simulink model "iter_imas_contr_4"  (Simulink 8.5)
settings: Solver=ode1  StartTime=EqTime  StopTime=1e8  FixedStep=SimStep  MaxStep=5.e-3  MinStep=2e-4  RelTol=1.e-3
undefined symbols (not defined in the file): Elong, g1, g1_term, g2, g2_term, g3, g3_term, g4, g4_term, g5, g5_term, g6, g6_term, Imax, key_imas, n_gaps, n_mc, ncam, npf, ntur, RupRd, scr_data, SimStep, Vcspf_up, vec_imas, volt
libraries: simulink x56
(part 1 of 3)
settings Model: Creator=Kavin  ModifiedByFormat=Kavin  LastModifiedBy=Kavin  ExtModeTrigMode=oneshot  ExtModeArmWhenConnect=off  ExtModeAutoUpdateStatusClock=off
settings DataIOCC: LimitDataPoints=off  TimeSaveName=sim_time  SignalLoggingName=sigsOut
settings OptimizationCC: BooleanDataType=off  OptimizeBlockIOStorage=off  BufferReuse=off  GlobalBufferReuse=off  ExpressionFolding=off  ExpressionDepthLimit=128  LocalBlockOutputs=off  InitFltsAndDblsToZero=on
settings DebuggingCC: SaveWithParameterizedLinksMsg=none  SignalResolutionControl=TryResolveAllWithWarning  MultiTaskDSMMsg=warning  MultiTaskCondExecSysMsg=none  FcnCallInpInsideContextMsg=UseLocalSettings  StateNameClashWarn=none
settings HardwareCC: TargetUnknown=on
settings CodeAppCC: IgnoreCustomStorageClasses=off
settings GRTTargetCC: TargetFcnLib=ansi_tfl_tmw.mat

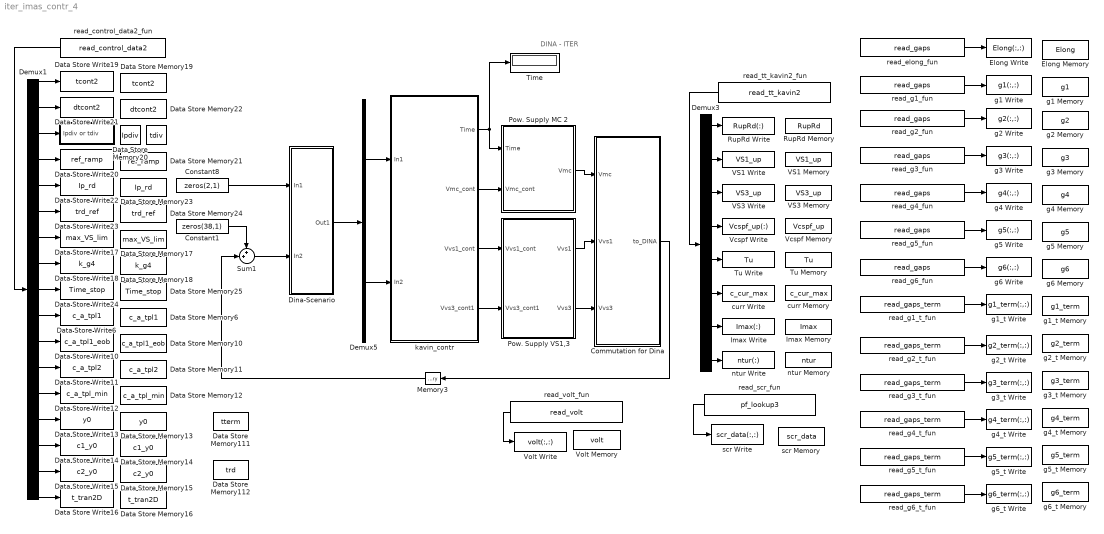
== system iter_imas_contr_4 ==
  note: DINA - ITER
  " " : DataStoreMemory  DataStoreName=tdiv  ReadBeforeWriteMsg=warning  WriteAfterWriteMsg=warning  WriteAfterReadMsg=warning  InitialValue=1e3
  "  " : Subsystem
  Commutation for Dina : Subsystem
  Constant1 : Constant  Value=zeros(38,1)
  Constant8 : Constant  Value=zeros(2,1)
  Data Store Memory10 : DataStoreMemory  DataStoreName=c_a_tpl1_eob  ReadBeforeWriteMsg=warning  WriteAfterWriteMsg=warning  WriteAfterReadMsg=warning
  Data Store Memory11 : DataStoreMemory  DataStoreName=c_a_tpl2  ReadBeforeWriteMsg=warning  WriteAfterWriteMsg=warning  WriteAfterReadMsg=warning
  Data Store Memory111 : DataStoreMemory  DataStoreName=tterm  ReadBeforeWriteMsg=warning  WriteAfterWriteMsg=warning  WriteAfterReadMsg=warning  InitialValue=1000
  Data Store Memory112 : DataStoreMemory  DataStoreName=trd  ReadBeforeWriteMsg=warning  WriteAfterWriteMsg=warning  WriteAfterReadMsg=warning  InitialValue=1000
  Data Store Memory12 : DataStoreMemory  DataStoreName=c_a_tpl_min  ReadBeforeWriteMsg=warning  WriteAfterWriteMsg=warning  WriteAfterReadMsg=warning
  Data Store Memory13 : DataStoreMemory  DataStoreName=y0  ReadBeforeWriteMsg=warning  WriteAfterWriteMsg=warning  WriteAfterReadMsg=warning
  Data Store Memory14 : DataStoreMemory  DataStoreName=c1_y0  ReadBeforeWriteMsg=warning  WriteAfterWriteMsg=warning  WriteAfterReadMsg=warning
  Data Store Memory15 : DataStoreMemory  DataStoreName=c2_y0  ReadBeforeWriteMsg=warning  WriteAfterWriteMsg=warning  WriteAfterReadMsg=warning
  Data Store Memory16 : DataStoreMemory  DataStoreName=t_tran2D  ReadBeforeWriteMsg=warning  WriteAfterWriteMsg=warning  WriteAfterReadMsg=warning
  Data Store Memory17 : DataStoreMemory  DataStoreName=max_VS_lim  ReadBeforeWriteMsg=warning  WriteAfterWriteMsg=warning  WriteAfterReadMsg=warning
  Data Store Memory18 : DataStoreMemory  DataStoreName=k_g4  ReadBeforeWriteMsg=warning  WriteAfterWriteMsg=warning  WriteAfterReadMsg=warning
  Data Store Memory19 : DataStoreMemory  DataStoreName=tcont2  ReadBeforeWriteMsg=warning  WriteAfterWriteMsg=warning  WriteAfterReadMsg=warning
  Data Store Memory20 : DataStoreMemory  DataStoreName=Ipdiv  ReadBeforeWriteMsg=warning  WriteAfterWriteMsg=warning  WriteAfterReadMsg=warning  InitialValue=0.1
  Data Store Memory21 : DataStoreMemory  DataStoreName=ref_ramp  ReadBeforeWriteMsg=warning  WriteAfterWriteMsg=warning  WriteAfterReadMsg=warning  InitialValue=1e-3
  Data Store Memory22 : DataStoreMemory  DataStoreName=dtcont2  ReadBeforeWriteMsg=warning  WriteAfterWriteMsg=warning  WriteAfterReadMsg=warning  InitialValue=1e-3
  Data Store Memory23 : DataStoreMemory  DataStoreName=Ip_rd  ReadBeforeWriteMsg=warning  WriteAfterWriteMsg=warning  WriteAfterReadMsg=warning
  Data Store Memory24 : DataStoreMemory  DataStoreName=trd_ref  ReadBeforeWriteMsg=warning  WriteAfterWriteMsg=warning  WriteAfterReadMsg=warning
  Data Store Memory25 : DataStoreMemory  DataStoreName=Time_stop  ReadBeforeWriteMsg=warning  WriteAfterWriteMsg=warning  WriteAfterReadMsg=warning
  Data Store Memory6 : DataStoreMemory  DataStoreName=c_a_tpl1  ReadBeforeWriteMsg=warning  WriteAfterWriteMsg=warning  WriteAfterReadMsg=warning
  Data Store Write10 : DataStoreWrite  DataStoreName=c_a_tpl1_eob  DataStoreElements=c_a_tpl1_eob
  Data Store Write11 : DataStoreWrite  DataStoreName=c_a_tpl2  DataStoreElements=c_a_tpl2
  Data Store Write12 : DataStoreWrite  DataStoreName=c_a_tpl_min  DataStoreElements=c_a_tpl_min
  Data Store Write13 : DataStoreWrite  DataStoreName=y0  DataStoreElements=y0
  Data Store Write14 : DataStoreWrite  DataStoreName=c1_y0  DataStoreElements=c1_y0
  Data Store Write15 : DataStoreWrite  DataStoreName=c2_y0  DataStoreElements=c2_y0
  Data Store Write16 : DataStoreWrite  DataStoreName=t_tran2D  DataStoreElements=t_tran2D
  Data Store Write17 : DataStoreWrite  DataStoreName=max_VS_lim  DataStoreElements=max_VS_lim
  Data Store Write18 : DataStoreWrite  DataStoreName=k_g4  DataStoreElements=k_g4
  Data Store Write19 : DataStoreWrite  DataStoreName=tcont2  DataStoreElements=tcont2
  Data Store Write20 : DataStoreWrite  DataStoreName=ref_ramp  DataStoreElements=ref_ramp
  Data Store Write21 : DataStoreWrite  DataStoreName=dtcont2  DataStoreElements=dtcont2
  Data Store Write22 : DataStoreWrite  DataStoreName=Ip_rd  DataStoreElements=Ip_rd
  Data Store Write23 : DataStoreWrite  DataStoreName=trd_ref  DataStoreElements=trd_ref
  Data Store Write24 : DataStoreWrite  DataStoreName=Time_stop  DataStoreElements=Time_stop
  Data Store Write6 : DataStoreWrite  DataStoreName=c_a_tpl1  DataStoreElements=c_a_tpl1
  Demux1 : Demux  Outputs=ones(1,17)
  Demux3 : Demux  Outputs=[6 1 1 11 1 1 11 12]
  Demux5 : Demux  Outputs=[15 123]
  Dina-Scenario : Subsystem
  Elong Memory : DataStoreMemory  DataStoreName=Elong  ReadBeforeWriteMsg=warning  WriteAfterWriteMsg=warning  WriteAfterReadMsg=warning  InitialValue=[0:49;zeros(1,50)]
  Elong Write : DataStoreWrite  DataStoreName=Elong  DataStoreElements=Elong(:,:)
  Imax Memory : DataStoreMemory  DataStoreName=Imax  ReadBeforeWriteMsg=warning  WriteAfterWriteMsg=warning  WriteAfterReadMsg=warning  InitialValue=ones(1,11)*1e6
  Imax Write : DataStoreWrite  DataStoreName=Imax  DataStoreElements=Imax(:)
  Memory3 : Memory
  Pow. Supply MC 2 : Subsystem
  Pow. Supply VS1,3 : Subsystem
  RupRd Memory : DataStoreMemory  DataStoreName=RupRd  ReadBeforeWriteMsg=warning  WriteAfterWriteMsg=warning  WriteAfterReadMsg=warning  InitialValue=[1; ones(3,1)*1e-6; -1e6; 1e-6]
  RupRd Write : DataStoreWrite  DataStoreName=RupRd  DataStoreElements=RupRd(:)
  Sum1 : Sum  Inputs=++|  SaturateOnIntegerOverflow=on  InputSameDT=on  OutDataTypeStr=Inherit: Same as first input
  Time : Display
  Tu Memory : DataStoreMemory  DataStoreName=Tu  ReadBeforeWriteMsg=warning  WriteAfterWriteMsg=warning  WriteAfterReadMsg=warning
  Tu Write : DataStoreWrite  DataStoreName=Tu  DataStoreElements=Tu
  VS1 Memory : DataStoreMemory  DataStoreName=VS1_up  ReadBeforeWriteMsg=warning  WriteAfterWriteMsg=warning  WriteAfterReadMsg=warning
  VS1 Write : DataStoreWrite  DataStoreName=VS1_up  DataStoreElements=VS1_up
  VS3 Memory : DataStoreMemory  DataStoreName=VS3_up  ReadBeforeWriteMsg=warning  WriteAfterWriteMsg=warning  WriteAfterReadMsg=warning
  VS3 Write : DataStoreWrite  DataStoreName=VS3_up  DataStoreElements=VS3_up
  Vcspf Memory : DataStoreMemory  DataStoreName=Vcspf_up  ReadBeforeWriteMsg=warning  WriteAfterWriteMsg=warning  WriteAfterReadMsg=warning  InitialValue=zeros(11,1)
  Vcspf Write : DataStoreWrite  DataStoreName=Vcspf_up  DataStoreElements=Vcspf_up(:)
  Volt Memory : DataStoreMemory  DataStoreName=volt  ReadBeforeWriteMsg=warning  WriteAfterWriteMsg=warning  WriteAfterReadMsg=warning  InitialValue=[(0:499);zeros(19,500)]
  Volt Write : DataStoreWrite  DataStoreName=volt  DataStoreElements=volt(:,:)
  curr Memory : DataStoreMemory  DataStoreName=c_cur_max  ReadBeforeWriteMsg=warning  WriteAfterWriteMsg=warning  WriteAfterReadMsg=warning
  curr Write : DataStoreWrite  DataStoreName=c_cur_max  DataStoreElements=c_cur_max
  g1 Memory : DataStoreMemory  DataStoreName=g1  ReadBeforeWriteMsg=warning  WriteAfterWriteMsg=warning  WriteAfterReadMsg=warning  InitialValue=[0:49;zeros(1,50)]
  g1 Write : DataStoreWrite  DataStoreName=g1  DataStoreElements=g1(:,:)
  g1_t Memory : DataStoreMemory  DataStoreName=g1_term  ReadBeforeWriteMsg=warning  WriteAfterWriteMsg=warning  WriteAfterReadMsg=warning  InitialValue=zeros(2, 50)
  g1_t Write : DataStoreWrite  DataStoreName=g1_term  DataStoreElements=g1_term(:,:)
  g2 Memory : DataStoreMemory  DataStoreName=g2  ReadBeforeWriteMsg=warning  WriteAfterWriteMsg=warning  WriteAfterReadMsg=warning  InitialValue=[0:49;zeros(1,50)]
  g2 Write : DataStoreWrite  DataStoreName=g2  DataStoreElements=g2(:,:)
  g2_t Memory : DataStoreMemory  DataStoreName=g2_term  ReadBeforeWriteMsg=warning  WriteAfterWriteMsg=warning  WriteAfterReadMsg=warning  InitialValue=zeros(2, 50)
  g2_t Write : DataStoreWrite  DataStoreName=g2_term  DataStoreElements=g2_term(:,:)
  g3 Memory : DataStoreMemory  DataStoreName=g3  ReadBeforeWriteMsg=warning  WriteAfterWriteMsg=warning  WriteAfterReadMsg=warning  InitialValue=[0:49;zeros(1,50)]
  g3 Write : DataStoreWrite  DataStoreName=g3  DataStoreElements=g3(:,:)
  g3_t Memory : DataStoreMemory  DataStoreName=g3_term  ReadBeforeWriteMsg=warning  WriteAfterWriteMsg=warning  WriteAfterReadMsg=warning  InitialValue=zeros(2, 50)
  g3_t Write : DataStoreWrite  DataStoreName=g3_term  DataStoreElements=g3_term(:,:)
  g4 Memory : DataStoreMemory  DataStoreName=g4  ReadBeforeWriteMsg=warning  WriteAfterWriteMsg=warning  WriteAfterReadMsg=warning  InitialValue=[0:49;zeros(1,50)]
  g4 Write : DataStoreWrite  DataStoreName=g4  DataStoreElements=g4(:,:)
  g4_t Memory : DataStoreMemory  DataStoreName=g4_term  ReadBeforeWriteMsg=warning  WriteAfterWriteMsg=warning  WriteAfterReadMsg=warning  InitialValue=zeros(2, 50)
  g4_t Write : DataStoreWrite  DataStoreName=g4_term  DataStoreElements=g4_term(:,:)
  g5 Memory : DataStoreMemory  DataStoreName=g5  ReadBeforeWriteMsg=warning  WriteAfterWriteMsg=warning  WriteAfterReadMsg=warning  InitialValue=[0:49;zeros(1,50)]
  g5 Write : DataStoreWrite  DataStoreName=g5  DataStoreElements=g5(:,:)
  g5_t Memory : DataStoreMemory  DataStoreName=g5_term  ReadBeforeWriteMsg=warning  WriteAfterWriteMsg=warning  WriteAfterReadMsg=warning  InitialValue=zeros(2, 50)
  g5_t Write : DataStoreWrite  DataStoreName=g5_term  DataStoreElements=g5_term(:,:)
  g6 Memory : DataStoreMemory  DataStoreName=g6  ReadBeforeWriteMsg=warning  WriteAfterWriteMsg=warning  WriteAfterReadMsg=warning  InitialValue=[0:49;zeros(1,50)]
  g6 Write : DataStoreWrite  DataStoreName=g6  DataStoreElements=g6(:,:)
  g6_t Memory : DataStoreMemory  DataStoreName=g6_term  ReadBeforeWriteMsg=warning  WriteAfterWriteMsg=warning  WriteAfterReadMsg=warning  InitialValue=zeros(2, 50)
  g6_t Write : DataStoreWrite  DataStoreName=g6_term  DataStoreElements=g6_term(:,:)
  kavin_contr : Subsystem
  ntur Memory : DataStoreMemory  DataStoreName=ntur  ReadBeforeWriteMsg=warning  WriteAfterWriteMsg=warning  WriteAfterReadMsg=warning  InitialValue="[554,554,554,554,554  248.6 115.2 185.9 169.9 216.8  459.4 1]"
  ntur Write : DataStoreWrite  DataStoreName=ntur  DataStoreElements=ntur(:)
  read_control_data2_fun : S-Function  FunctionName=read_control_data2  SFunctionModules=read_control_data2_wrapper read_control_data2
  read_elong_fun : S-Function  FunctionName=read_gaps  Parameters=0  SFunctionModules='read_gaps_wrapper read_gaps'
  read_g1_fun : S-Function  FunctionName=read_gaps  Parameters=1  SFunctionModules='read_gaps_wrapper read_gaps'
  read_g1_t_fun : S-Function  FunctionName=read_gaps_term  Parameters=1  SFunctionModules='read_gaps_term_wrapper read_gaps_term'
  read_g2_fun : S-Function  FunctionName=read_gaps  Parameters=2  SFunctionModules='read_gaps_wrapper read_gaps'
  read_g2_t_fun : S-Function  FunctionName=read_gaps_term  Parameters=2  SFunctionModules='read_gaps_term_wrapper read_gaps_term'
  read_g3_fun : S-Function  FunctionName=read_gaps  Parameters=3  SFunctionModules='read_gaps_wrapper read_gaps'
  read_g3_t_fun : S-Function  FunctionName=read_gaps_term  Parameters=3  SFunctionModules='read_gaps_term_wrapper read_gaps_term'
  read_g4_fun : S-Function  FunctionName=read_gaps  Parameters=4  SFunctionModules='read_gaps_wrapper read_gaps'
  read_g4_t_fun : S-Function  FunctionName=read_gaps_term  Parameters=4  SFunctionModules='read_gaps_term_wrapper read_gaps_term'
  read_g5_fun : S-Function  FunctionName=read_gaps  Parameters=5  SFunctionModules='read_gaps_wrapper read_gaps'
  read_g5_t_fun : S-Function  FunctionName=read_gaps_term  Parameters=5  SFunctionModules='read_gaps_term_wrapper read_gaps_term'
  read_g6_fun : S-Function  FunctionName=read_gaps  Parameters=6  SFunctionModules='read_gaps_wrapper read_gaps'
  read_g6_t_fun : S-Function  FunctionName=read_gaps_term  Parameters=6  SFunctionModules='read_gaps_term_wrapper read_gaps_term'
  read_scr_fun : S-Function  FunctionName=pf_lookup3  Parameters=1  SFunctionModules='pf_lookup3_wrapper read_pf'
  read_tt_kavin2_fun : S-Function  FunctionName=read_tt_kavin2  SFunctionModules=read_tt_kavin2_wrapper read_tt_kavin2
  read_volt_fun : S-Function  FunctionName=read_volt  Parameters=12  SFunctionModules='read_volt_wrapper read_volt'
  scr Memory : DataStoreMemory  DataStoreName=scr_data  ReadBeforeWriteMsg=warning  WriteAfterWriteMsg=warning  WriteAfterReadMsg=warning  InitialValue=[(0:499); zeros(12,500)]
  scr Write : DataStoreWrite  DataStoreName=scr_data  DataStoreElements=scr_data(:,:)
  wires:
  Demux5/1 -> kavin_contr/1(In1)
  Demux5/2 -> kavin_contr/2(In2)
  Dina-Scenario/1(Out1) -> Demux5/1
  Constant8/1 -> Dina-Scenario/1(In1)
  Constant1/1 -> Sum1/1
  Sum1/1 -> Dina-Scenario/2(In2)
  kavin_contr/2(Vmc_cont) -> Pow. Supply MC 2/2(Vmc_cont)
  Pow. Supply MC 2/1(Vmc) -> Commutation for Dina/1(Vmc)
  Commutation for Dina/1(to_DINA) -> Memory3/1
  read_tt_kavin2_fun/1 -> Demux3/1
  kavin_contr/3(Vvs1_cont) -> Pow. Supply VS1,3/1(Vvs1_cont)
  kavin_contr/4(Vvs3_cont1) -> Pow. Supply VS1,3/2(Vvs3_cont1)
  Pow. Supply VS1,3/2(Vvs3) -> Commutation for Dina/3(Vvs3)
  Pow. Supply VS1,3/1(Vvs1) -> Commutation for Dina/2(Vvs1)
  Demux3/8 -> ntur Write/1
  Demux3/7 -> Imax Write/1
  Demux3/6 -> curr Write/1
  Demux3/5 -> Tu Write/1
  Demux3/4 -> Vcspf Write/1
  Demux3/3 -> VS3 Write/1
  Demux3/2 -> VS1 Write/1
  Demux3/1 -> RupRd Write/1
  Memory3/1 -> Sum1/2
  read_elong_fun/1 -> Elong Write/1
  read_g1_fun/1 -> g1 Write/1
  read_g2_fun/1 -> g2 Write/1
  read_g3_fun/1 -> g3 Write/1
  read_g4_fun/1 -> g4 Write/1
  read_g5_fun/1 -> g5 Write/1
  read_g6_fun/1 -> g6 Write/1
  read_g1_t_fun/1 -> g1_t Write/1
  read_g2_t_fun/1 -> g2_t Write/1
  read_g3_t_fun/1 -> g3_t Write/1
  read_g4_t_fun/1 -> g4_t Write/1
  read_g5_t_fun/1 -> g5_t Write/1
  read_g6_t_fun/1 -> g6_t Write/1
  read_scr_fun/1 -> scr Write/1
  kavin_contr/1(Time) -> Time/1, Pow. Supply MC 2/1(Time)
  read_volt_fun/1 -> Volt Write/1
  read_control_data2_fun/1 -> Demux1/1
  Demux1/6 -> Data Store Write23/1
  Demux1/5 -> Data Store Write22/1
  Demux1/4 -> Data Store Write20/1
  Demux1/3 -> "  "/1("Ipdiv or tdiv ")
  Demux1/2 -> Data Store Write21/1
  Demux1/1 -> Data Store Write19/1
  Demux1/9 -> Data Store Write24/1
  Demux1/10 -> Data Store Write6/1
  Demux1/11 -> Data Store Write10/1
  Demux1/12 -> Data Store Write11/1
  Demux1/13 -> Data Store Write12/1
  Demux1/14 -> Data Store Write13/1
  Demux1/15 -> Data Store Write14/1
  Demux1/16 -> Data Store Write15/1
  Demux1/17 -> Data Store Write16/1
  Demux1/7 -> Data Store Write17/1
  Demux1/8 -> Data Store Write18/1

== system iter_imas_contr_4/   ==
  "Ipdiv or tdiv " : Inport
  Data Store Write19 : DataStoreWrite  DataStoreName=Ipdiv
  If : If  IfExpression=u1 >= 0  ShowElse=off
  If Action : Subsystem  TreatAsAtomicUnit=on
  wires:
  "Ipdiv or tdiv "/1 -> Data Store Write19/1, If Action/1("tdiv "), If/1
  If/1 -> If Action/Action

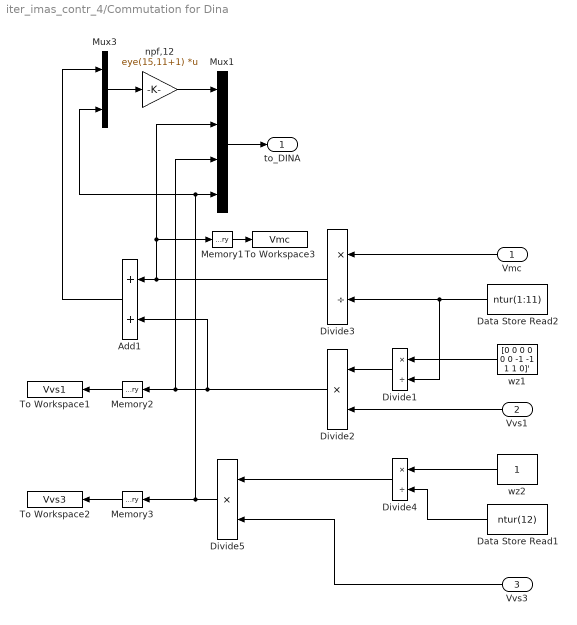
== system iter_imas_contr_4/Commutation for Dina ==
  Vmc : Inport
  Vvs1 : Inport  Port=2
  Vvs3 : Inport  Port=3
  Add1 : Sum
  Data Store Read1 : DataStoreRead  DataStoreName=ntur  DataStoreElements=ntur(12)
  Data Store Read2 : DataStoreRead  DataStoreName=ntur  DataStoreElements=ntur(1:11)
  Divide1 : Product  Inputs=*/
  Divide2 : Product  Inputs=**
  Divide3 : Product  Inputs=*/
  Divide4 : Product  Inputs=*/
  Divide5 : Product  Inputs=**
  Memory1 : Memory
  Memory2 : Memory
  Memory3 : Memory
  Mux1 : Mux
  Mux3 : Mux  Inputs=2
  To Workspace1 : ToWorkspace  VariableName=Vvs1
  To Workspace2 : ToWorkspace  VariableName=Vvs3
  To Workspace3 : ToWorkspace  VariableName=Vmc
  npf,12 : Gain  Gain=eye(15,11+1)  Multiplication=Matrix(K*u)
  wz1 : Constant  Value=[0 0 0 0 0 0 -1 -1 1 1 0]'
  wz2 : Constant
  to_DINA : Outport
  wires:
  Divide2/1 -> Add1/2, Mux1/3, Memory2/1
  Mux1/1 -> to_DINA/1
  Add1/1 -> Mux3/1
  Mux3/1 -> npf,12/1
  npf,12/1 -> Mux1/1
  Divide3/1 -> Add1/1, Mux1/2, Memory1/1
  Vmc/1 -> Divide3/1
  Data Store Read2/1 -> Divide1/2, Divide3/2
  wz1/1 -> Divide1/1
  Divide1/1 -> Divide2/1
  Vvs1/1 -> Divide2/2
  wz2/1 -> Divide4/1
  Data Store Read1/1 -> Divide4/2
  Divide4/1 -> Divide5/1
  Vvs3/1 -> Divide5/2
  Divide5/1 -> Mux3/2, Mux1/4, Memory3/1
  Memory1/1 -> To Workspace3/1
  Memory2/1 -> To Workspace1/1
  Memory3/1 -> To Workspace2/1

== system iter_imas_contr_4/Dina-Scenario ==
  In1 : Inport
  In2 : Inport  Port=2
  Constant15 : Constant  Value=zeros(54,1)
  Mux2 : Mux  Inputs=2
  S-Function1 : S-Function  FunctionName=dina_imas  Parameters=key_imas,vec_imas
  Terminator3 : Terminator
  To Workspace21 : ToWorkspace  VariableName=sim_shape
      settings: Decimation=DecimShape
  Out1 : Outport
  wires:
  In1/1 -> S-Function1/1
  S-Function1/2 -> Mux2/2
  S-Function1/3 -> To Workspace21/1
  S-Function1/4 -> Terminator3/1
  S-Function1/1 -> Mux2/1
  Mux2/1 -> Out1/1
  In2/1 -> S-Function1/2
  Constant15/1 -> S-Function1/3

== system iter_imas_contr_4/Pow. Supply MC 2 ==
  Time : Inport
  Vmc_cont : Inport  Port=2
  Difference : simulink/Discrete/Difference  ICPrevInput=0.0  InputProcessing=Inherited  OutMin=[]  OutMax=[]  OutDataType=sfix(16)  OutScaling=2^-10  DoSatur=off
  Pow. Supply MC 1 : Subsystem
  Vmc : Outport
  wires:
  Time/1 -> Difference/1
  Difference/1 -> Pow. Supply MC 1/1(dt)
  Pow. Supply MC 1/1(Vmc) -> Vmc/1
  Vmc_cont/1 -> Pow. Supply MC 1/2(Vmc_cont)

== system iter_imas_contr_4/Pow. Supply VS1,3 ==
  Vvs1_cont : Inport
  Vvs3_cont1 : Inport  Port=2
  Data Store Read1 : DataStoreRead  DataStoreName=VS1_up  DataStoreElements=VS1_up
  Data Store Read3 : DataStoreRead  DataStoreName=VS3_up  DataStoreElements=VS3_up
  Gain : Gain  Gain=-1
  Gain1 : Gain  Gain=-1
  Saturation Dynamic : simulink/Discontinuities/Saturation Dynamic  OutMin=[]  OutMax=[]  OutDataTypeStr=Inherit: Same as second input  OutDataType=fixdt(1, 16)  OutScaling=2^-10  DoSatur=off
  Saturation Dynamic1 : simulink/Discontinuities/Saturation Dynamic  OutMin=[]  OutMax=[]  OutDataTypeStr=Inherit: Same as second input  OutDataType=fixdt(1, 16)  OutScaling=2^-10  DoSatur=off
  Vvs1 : Outport
  Vvs3 : Outport  Port=2
  wires:
  Data Store Read1/1 -> Gain/1, Saturation Dynamic/1
  Gain/1 -> Saturation Dynamic/3
  Vvs1_cont/1 -> Saturation Dynamic/2
  Gain1/1 -> Saturation Dynamic1/3
  Data Store Read3/1 -> Gain1/1, Saturation Dynamic1/1
  Vvs3_cont1/1 -> Saturation Dynamic1/2
  Saturation Dynamic/1 -> Vvs1/1
  Saturation Dynamic1/1 -> Vvs3/1

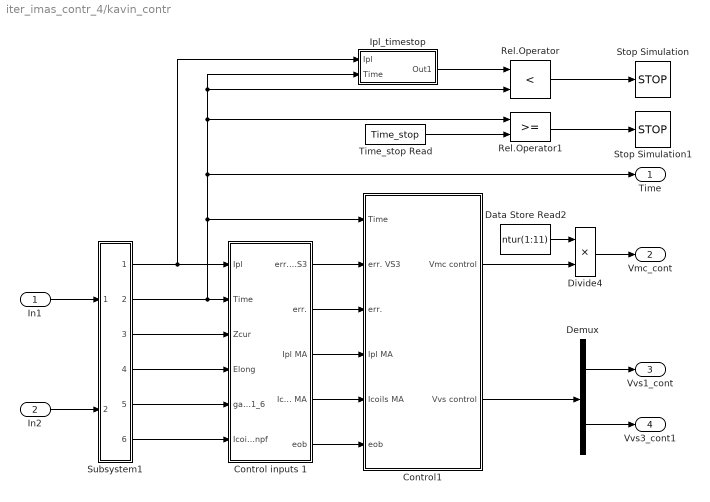
== system iter_imas_contr_4/kavin_contr ==
  In1 : Inport
  In2 : Inport  Port=2
  Control inputs 1 : Subsystem  Priority=1
  Control1 : Subsystem  Priority=2
  Data Store Read2 : DataStoreRead  DataStoreName=ntur  DataStoreElements=ntur(1:11)
  Demux : Demux  Outputs=2
  Divide4 : Product  Inputs=**
  Ipl_timestop : Subsystem
  Rel.Operator : RelationalOperator  Operator=<  OutDataTypeStr=boolean
  Rel.Operator1 : RelationalOperator  OutDataTypeStr=boolean
  Stop Simulation : Stop
  Stop Simulation1 : Stop
  Subsystem1 : Subsystem
  Time_stop Read : DataStoreRead  DataStoreName=Time_stop  DataStoreElements=Time_stop
  Time : Outport
  Vmc_cont : Outport  Port=2
  Vvs1_cont : Outport  Port=3
  Vvs3_cont1 : Outport  Port=4
  wires:
  Control inputs 1/2(err.) -> Control1/3(err.)
  Control inputs 1/4(Icoils MA) -> Control1/5(Icoils MA)
  Rel.Operator/1 -> Stop Simulation/1
  Rel.Operator1/1 -> Stop Simulation1/1
  Time_stop Read/1 -> Rel.Operator1/2
  Control1/2(Vvs control) -> Demux/1
  Demux/1 -> Vvs1_cont/1
  Demux/2 -> Vvs3_cont1/1
  Divide4/1 -> Vmc_cont/1
  Control1/1(Vmc control) -> Divide4/2
  Data Store Read2/1 -> Divide4/1
  Control inputs 1/1(err. VS3) -> Control1/2(err. VS3)
  Control inputs 1/3(Ipl MA) -> Control1/4(Ipl MA)
  Control inputs 1/5(eob) -> Control1/6(eob)
  Subsystem1/2("time ") -> Control1/1(Time), Ipl_timestop/2(Time), Rel.Operator/2, Rel.Operator1/1, Time/1, Control inputs 1/2(Time)
  Subsystem1/1(Ipl) -> Control inputs 1/1(Ipl), Ipl_timestop/1(Ipl)
  In1/1 -> Subsystem1/1("  ")
  In2/1 -> Subsystem1/2(" ")
  Subsystem1/3(Zcurr) -> Control inputs 1/3(Zcur)
  Subsystem1/4(Elong) -> Control inputs 1/4(Elong)
  Subsystem1/5(gaps) -> Control inputs 1/5(gaps1_6)
  Subsystem1/6(Icoil1) -> Control inputs 1/6(Icoil1_npf)
  Ipl_timestop/1(Out1) -> Rel.Operator/1

== system iter_imas_contr_4/  /If Action ==
  "tdiv " : Inport
  Action Port : ActionPort  ActionType=then
  Data Store Write19 : DataStoreWrite  DataStoreName=tdiv
  wires:
  "tdiv "/1 -> Data Store Write19/1

== system iter_imas_contr_4/Pow. Supply MC 2/Pow. Supply MC 1 ==
  dt : Inport
  Vmc_cont : Inport  Port=2
  Add1 : Sum  Inputs=-+
  Add2 : Sum
  Divide : Product  Inputs=*/
  Divide1 : Product  Inputs=**
  MC rate : Subsystem
  MC satur. : Subsystem
  Memory1 : Memory
  To Workspace1 : ToWorkspace  VariableName=Vcont1  SampleTime=-1
  Vmc : Outport
  wires:
  dt/1 -> Divide/2, Divide1/2
  Add1/1 -> Divide/1
  Vmc_cont/1 -> Add1/2
  Divide1/1 -> Add2/2
  Memory1/1 -> Add2/1, Add1/1
  MC satur./1(Out1) -> To Workspace1/1, Memory1/1, Vmc/1
  Add2/1 -> MC satur./1(In1)
  Divide/1 -> MC rate/1(In1)
  MC rate/1(Out1) -> Divide1/1

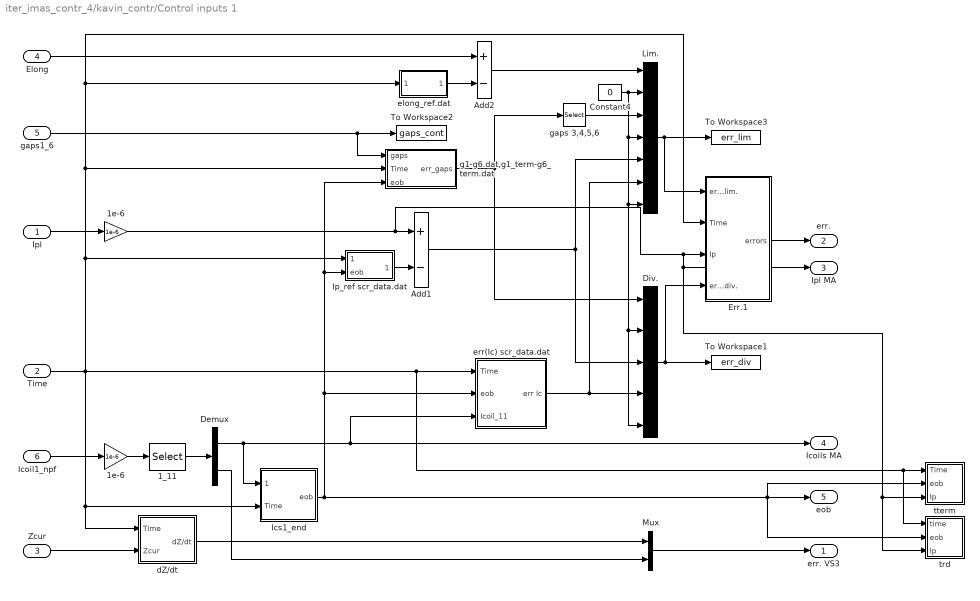
== system iter_imas_contr_4/kavin_contr/Control inputs 1 ==
  Ipl : Inport
  Time : Inport  Port=2
  Zcur : Inport  Port=3
  Elong : Inport  Port=4
  gaps1_6 : Inport  Port=5
  Icoil1_npf : Inport  Port=6
  1_11 : Selector  InputPortWidth=15  Indices=[1:11+1]
  1e-6 : Gain  Gain=1e-6
  "1e-6   " : Gain  Gain=1e-6
  Add1 : Sum  Inputs=+-
  Add2 : Sum  Inputs=+-
  Constant4 : Constant  Value=0  VectorParams1D=off
  Demux : Demux  Outputs=[11 1]
  "Div. " : Mux  Inputs=5
  Err.1 : Subsystem
  Ics1_end : Subsystem
  Ip_ref scr_data.dat : Subsystem
  "Lim. " : Mux  Inputs=7
  Mux : Mux  Inputs=2
  To Workspace1 : ToWorkspace  VariableName=err_div
  To Workspace2 : ToWorkspace  VariableName=gaps_cont
  To Workspace3 : ToWorkspace  VariableName=err_lim
  dZ/dt : Subsystem
  elong_ref.dat : Subsystem
  err(Ic) scr_data.dat : Subsystem
  g1-g6.dat,g1_term-g6_term.dat : Subsystem
  gaps 3,4,5,6 : Selector  InputPortWidth=6  Indices=[3:6]
  trd : Subsystem
  tterm : Subsystem
  err. VS3 : Outport
  err. : Outport  Port=2
  Ipl MA : Outport  Port=3
  Icoils MA : Outport  Port=4
  eob : Outport  Port=5
  wires:
  Zcur/1 -> dZ/dt/2(Zcur)
  gaps1_6/1 -> g1-g6.dat,g1_term-g6_term.dat/1(gaps), To Workspace2/1
  Ipl/1 -> 1e-6/1
  Icoil1_npf/1 -> "1e-6   "/1
  "1e-6   "/1 -> 1_11/1
  1_11/1 -> Demux/1
  Elong/1 -> Add2/1
  Ip_ref scr_data.dat/1(Ip ref) -> Add1/2
  1e-6/1 -> Add1/1, tterm/3(Ip), trd/3(Ip), Ipl MA/1, Err.1/3(Ip)
  Demux/1 -> Ics1_end/1(Icoils,MA), Icoils MA/1, err(Ic) scr_data.dat/3(Icoil_11)
  Add2/1 -> "Lim. "/1
  Constant4/1 -> "Div. "/5, "Div. "/2, "Lim. "/7, "Lim. "/4, "Lim. "/2
  Add1/1 -> "Lim. "/5, "Div. "/3
  err(Ic) scr_data.dat/1(err Ic) -> "Div. "/4, "Lim. "/6
  g1-g6.dat,g1_term-g6_term.dat/1(err_gaps) -> gaps 3,4,5,6/1, "Div. "/1
  Demux/2 -> Mux/2
  Mux/1 -> err. VS3/1
  "Div. "/1 -> To Workspace1/1, Err.1/4(err. div.)
  "Lim. "/1 -> To Workspace3/1, Err.1/1(err. lim.)
  Err.1/1(errors) -> err./1
  elong_ref.dat/1(Elong) -> Add2/2
  dZ/dt/1(dZ/dt) -> Mux/1
  Time/1 -> dZ/dt/1(Time), Ics1_end/2(Time), Err.1/2(Time), elong_ref.dat/1(Time), g1-g6.dat,g1_term-g6_term.dat/2(Time), Ip_ref scr_data.dat/1(Time), trd/1(time), tterm/1(Time), err(Ic) scr_data.dat/1(Time)
  Ics1_end/1(eob) -> trd/2(eob), tterm/2(eob), eob/1, g1-g6.dat,g1_term-g6_term.dat/3(eob), Ip_ref scr_data.dat/2(eob), err(Ic) scr_data.dat/2(eob)
  gaps 3,4,5,6/1 -> "Lim. "/3

== system iter_imas_contr_4/kavin_contr/Control1 ==
  Time : Inport
  err. VS3 : Inport  Port=2
  err. : Inport  Port=3
  Ipl MA : Inport  Port=4
  Icoils MA : Inport  Port=5
  eob : Inport  Port=6
  Curr. satur.1 : Subsystem
  Data Store Read1 : DataStoreRead  DataStoreName=Imax  DataStoreElements=Imax(:)
  Sum : Subsystem
  VS control : Subsystem
  controllers : Subsystem
  volt.dat : Subsystem
  Vmc control : Outport
  Vvs control : Outport  Port=2
  wires:
  VS control/1(Vvs) -> Vvs control/1
  Icoils MA/1 -> controllers/1(Icoils), Curr. satur.1/1(Ic)
  Curr. satur.1/1(Volt. curr. satur.) -> Vmc control/1
  Data Store Read1/1 -> Curr. satur.1/3(Imax)
  err. VS3/1 -> VS control/1(VS3 err)
  err./1 -> controllers/2(err.)
  controllers/2(Div.contr) -> Sum/2(Div.contr.)
  controllers/1(lim.contr.) -> Sum/1(Lim.contr.)
  Sum/1("  ") -> Curr. satur.1/2(Vmc)
  volt.dat/1(volt) -> Sum/4(volt.dat)
  Time/1 -> controllers/3("Time "), VS control/2(Time), volt.dat/1(Time)
  Ipl MA/1 -> controllers/5(Ipl), VS control/4(Ipl)
  eob/1 -> controllers/4(eob), VS control/3(eob)
  controllers/3(Curr.term.contr) -> Sum/3(Curr. term. contr)

== system iter_imas_contr_4/kavin_contr/Ipl_timestop ==
  Ipl : Inport
  Time : Inport  Port=2
  -1 : Gain  Gain=-1
  Constant4 : Constant  Value=50  VectorParams1D=off
  "Ip<1e-4 " : Switch  Criteria=u2 > Threshold  Threshold=-1e-4
  Memory2 : Memory
  Sum2 : Sum
  Out1 : Outport
  wires:
  Sum2/1 -> Out1/1
  Memory2/1 -> "Ip<1e-4 "/1
  -1/1 -> "Ip<1e-4 "/2
  "Ip<1e-4 "/1 -> Memory2/1, Sum2/1
  Constant4/1 -> Sum2/2
  Time/1 -> "Ip<1e-4 "/3
  Ipl/1 -> -1/1

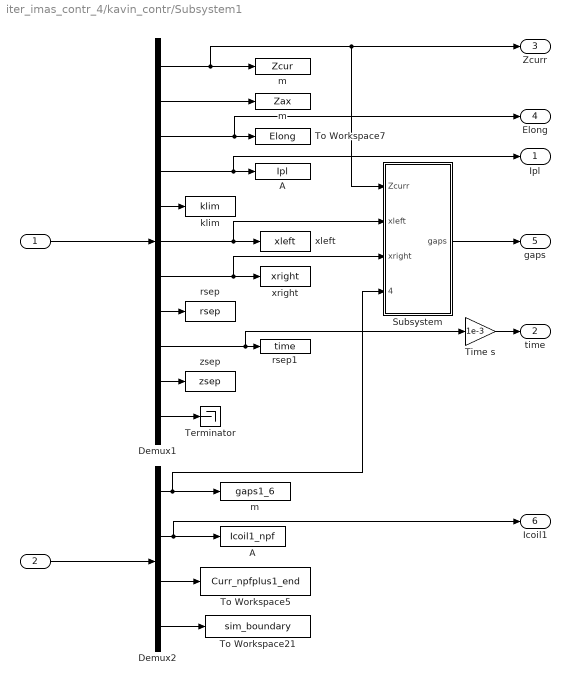
== system iter_imas_contr_4/kavin_contr/Subsystem1 ==
  "  " : Inport
  " " : Inport  Port=2
  A : ToWorkspace  VariableName=Ipl
  "A  " : ToWorkspace  VariableName=Icoil1_npf
  Demux1 : Demux  Outputs=[1 1 1 1 1 1 1 1 1 1 5 ]
  Demux2 : Demux  Outputs=[n_gaps npf ncam 2]
  Subsystem : Subsystem
  Terminator : Terminator
  Time s : Gain  Gain=1e-3
  To Workspace21 : ToWorkspace  VariableName=sim_boundary
      settings: Decimation=DecimShape
  To Workspace5 : ToWorkspace  VariableName=Curr_npfplus1_end
  To Workspace7 : ToWorkspace  VariableName=Elong
  klim : ToWorkspace  VariableName=klim
  m : ToWorkspace  VariableName=gaps1_6
  "m  " : ToWorkspace  VariableName=Zax
  "m   " : ToWorkspace  VariableName=Zcur
  rsep : ToWorkspace  VariableName=rsep
  rsep1 : ToWorkspace  VariableName=time
  xleft : ToWorkspace  VariableName=xleft
  xright : ToWorkspace  VariableName=xright
  zsep : ToWorkspace  VariableName=zsep
  Ipl : Outport
  "time " : Outport  Port=2
  Zcurr : Outport  Port=3
  Elong : Outport  Port=4
  gaps : Outport  Port=5
  Icoil1 : Outport  Port=6
  wires:
  Demux1/10 -> zsep/1
  Demux1/9 -> rsep1/1, Time s/1
  Time s/1 -> "time "/1
  Demux1/11 -> Terminator/1
  Subsystem/1(gaps) -> gaps/1
  Demux2/1 -> m/1, Subsystem/4(gaps1_6)
  Demux1/8 -> rsep/1
  Demux1/7 -> xright/1, Subsystem/3(xright)
  Demux1/6 -> xleft/1, Subsystem/2(xleft)
  Demux1/5 -> klim/1
  " "/1 -> Demux2/1
  "  "/1 -> Demux1/1
  Demux2/2 -> Icoil1/1, "A  "/1
  Demux2/3 -> To Workspace5/1
  Demux1/4 -> Ipl/1, A/1
  Demux2/4 -> To Workspace21/1
  Demux1/3 -> To Workspace7/1, Elong/1
  Demux1/1 -> Subsystem/1(Zcurr), Zcurr/1, "m   "/1
  Demux1/2 -> "m  "/1

== system iter_imas_contr_4/Pow. Supply MC 2/Pow. Supply MC 1/MC rate ==
  In1 : Inport
  -1 : Gain  Gain=-1
  2 : Gain  Gain=2
  Data Store Read1 : DataStoreRead  DataStoreName=Vcspf_up  DataStoreElements=Vcspf_up(:)
  Data Store Read3 : DataStoreRead  DataStoreName=Tu  DataStoreElements=Tu
  Divide1 : Product  Inputs=*/
  Saturation Dynamic : simulink/Discontinuities/Saturation Dynamic  OutMin=[]  OutMax=[]  OutDataTypeStr=Inherit: Same as second input  OutDataType=fixdt(1, 16)  OutScaling=2^-10  DoSatur=off
  Out1 : Outport
  wires:
  Saturation Dynamic/1 -> Out1/1
  In1/1 -> Saturation Dynamic/2
  Divide1/1 -> Saturation Dynamic/1, -1/1
  Data Store Read1/1 -> 2/1
  2/1 -> Divide1/1
  Data Store Read3/1 -> Divide1/2
  -1/1 -> Saturation Dynamic/3

== system iter_imas_contr_4/Pow. Supply MC 2/Pow. Supply MC 1/MC satur. ==
  In1 : Inport
  Data Store Read1 : DataStoreRead  DataStoreName=Vcspf_up  DataStoreElements=Vcspf_up(:)
  Gain : Gain  Gain=-1
  Saturation Dynamic : simulink/Discontinuities/Saturation Dynamic  OutMin=[]  OutMax=[]  OutDataTypeStr=Inherit: Same as second input  OutDataType=fixdt(1, 16)  OutScaling=2^-10  DoSatur=off
  Out1 : Outport
  wires:
  Data Store Read1/1 -> Gain/1, Saturation Dynamic/1
  Gain/1 -> Saturation Dynamic/3
  In1/1 -> Saturation Dynamic/2
  Saturation Dynamic/1 -> Out1/1

== system iter_imas_contr_4/kavin_contr/Control inputs 1/Err.1 ==
  err. lim. : Inport
  Time : Inport  Port=2
  Ip : Inport  Port=3
  err. div. : Inport  Port=4
  2 : Switch  Threshold=1
  3 : Switch
  Abs : Abs
  Data Store Read1 : DataStoreRead  DataStoreName=Ipdiv
  Data Store Read2 : DataStoreRead  DataStoreName=tdiv
  Relational Operator : RelationalOperator  OutDataTypeStr=float('double')
  Relational Operator1 : RelationalOperator  Operator=<=  OutDataTypeStr=float('double')
  Trigger : Subsystem
  "tdiv if Ip is set " : Subsystem
  errors : Outport
  wires:
  2/1 -> errors/1
  Data Store Read1/1 -> 3/2, "tdiv if Ip is set "/2("tIp_tr "), Abs/1
  Time/1 -> Relational Operator/1, "tdiv if Ip is set "/3(Time)
  Relational Operator/1 -> 3/1
  Relational Operator1/1 -> Trigger/1(Input)
  3/1 -> 2/2
  Data Store Read2/1 -> Relational Operator/2
  Trigger/1(State) -> 3/3, "tdiv if Ip is set "/1(1 or 0)
  Ip/1 -> Relational Operator1/2
  Abs/1 -> Relational Operator1/1
  err. div./1 -> 2/1
  err. lim./1 -> 2/3

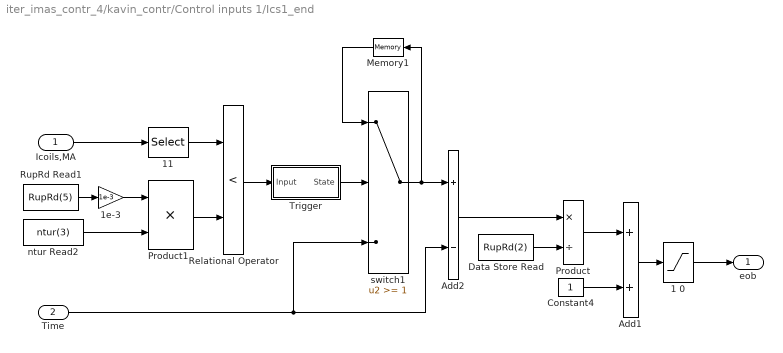
== system iter_imas_contr_4/kavin_contr/Control inputs 1/Ics1_end ==
  Icoils,MA : Inport
  Time : Inport  Port=2
  1 0 : Saturate  UpperLimit=1  LowerLimit=0
  11 : Selector  InputPortWidth=11  Indices=3
  1e-3 : Gain  Gain=1e-3
  Add1 : Sum
  Add2 : Sum  Inputs=+-
  Constant4 : Constant  VectorParams1D=off
  Data Store Read : DataStoreRead  DataStoreName=RupRd  DataStoreElements=RupRd(2)
  Memory1 : Memory
  Product : Product  Inputs=*/
  Product1 : Product  Inputs=**
  Relational Operator : RelationalOperator  Operator=<  OutDataTypeStr=float('double')
  RupRd Read1 : DataStoreRead  DataStoreName=RupRd  DataStoreElements=RupRd(5)
  Trigger : Subsystem
  ntur Read2 : DataStoreRead  DataStoreName=ntur  DataStoreElements=ntur(3)
  switch1 : Switch  Threshold=1
  eob : Outport
  wires:
  1 0/1 -> eob/1
  11/1 -> Relational Operator/1
  Icoils,MA/1 -> 11/1
  RupRd Read1/1 -> 1e-3/1
  1e-3/1 -> Product1/1
  ntur Read2/1 -> Product1/2
  Product1/1 -> Relational Operator/2
  Time/1 -> switch1/3, Add2/2
  switch1/1 -> Memory1/1, Add2/1
  Add2/1 -> Product/1
  Product/1 -> Add1/1
  Constant4/1 -> Add1/2
  Add1/1 -> 1 0/1
  Data Store Read/1 -> Product/2
  Trigger/1(State) -> switch1/2
  Relational Operator/1 -> Trigger/1(Input)
  Memory1/1 -> switch1/1

== system iter_imas_contr_4/kavin_contr/Control inputs 1/Ip_ref scr_data.dat ==
  Time : Inport
  eob : Inport  Port=2
  Divide6 : Product  Inputs=**
  Ipref : simulink/Lookup Tables/Lookup Table Dynamic  LookUpMeth=Interpolation-Use End Values  OutDataTypeStr=fixdt('double')  OutputDataTypeScalingMode=Specify via dialog  OutDataType=fixdt('double')  OutScaling=2^-10  DoSatur=off
  Memory1 : Memory
  c_eob : Switch  Threshold=1
  scr1 Read : DataStoreRead  DataStoreName=scr_data  DataStoreElements=scr_data(1,:)
  scr2 Read : DataStoreRead  DataStoreName=scr_data  DataStoreElements=scr_data(2,:)
  Ip ref : Outport
  wires:
  c_eob/1 -> Divide6/1, Memory1/1
  Divide6/1 -> Ip ref/1
  eob/1 -> c_eob/2, Divide6/2
  Memory1/1 -> c_eob/3
  scr2 Read/1 -> Ipref/3
  scr1 Read/1 -> Ipref/2
  Ipref/1 -> c_eob/1
  Time/1 -> Ipref/1

== system iter_imas_contr_4/kavin_contr/Control inputs 1/dZ/dt ==
  Time : Inport
  Zcur : Inport  Port=2
  Difference : simulink/Discrete/Difference  ICPrevInput=0.0  InputProcessing=Inherited  OutMin=[]  OutMax=[]  OutDataType=sfix(16)  OutScaling=2^-10  DoSatur=off
  Difference1 : simulink/Discrete/Difference  ICPrevInput=0  InputProcessing=Inherited  OutMin=[]  OutMax=[]  OutDataType=sfix(16)  OutScaling=2^-10  DoSatur=off
  Divide : Product  Inputs=*/
  dZ/dt : Outport
  wires:
  Zcur/1 -> Difference/1
  Time/1 -> Difference1/1
  Difference/1 -> Divide/1
  Difference1/1 -> Divide/2
  Divide/1 -> dZ/dt/1

== system iter_imas_contr_4/kavin_contr/Control inputs 1/elong_ref.dat ==
  Time : Inport
  Elong Read : DataStoreRead  DataStoreName=Elong
  Selector : Selector  NumberOfDimensions=2  InputPortWidth=13  IndexOptions=Index vector (dialog),Select all  Indices=2,1  OutputSizes=1,1
  Selector1 : Selector  NumberOfDimensions=2  InputPortWidth=13  IndexOptions=Index vector (dialog),Select all  Indices=1,1  OutputSizes=1,1
  elong : simulink/Lookup Tables/Lookup Table Dynamic  LookUpMeth=Interpolation-Use End Values  OutDataTypeStr=fixdt('double')  OutputDataTypeScalingMode=Specify via dialog  OutDataType=fixdt('double')  OutScaling=2^-10  DoSatur=off
  Elong : Outport
  wires:
  elong/1 -> Elong/1
  Selector/1 -> elong/3
  Selector1/1 -> elong/2
  Time/1 -> elong/1
  Elong Read/1 -> Selector/1, Selector1/1

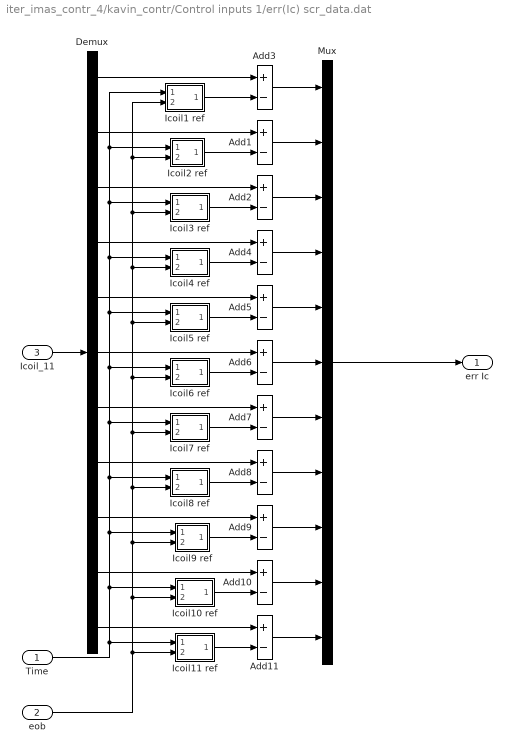
== system iter_imas_contr_4/kavin_contr/Control inputs 1/err(Ic) scr_data.dat ==
  Time : Inport
  eob : Inport  Port=2
  Icoil_11 : Inport  Port=3
  Add{1..11} (11 alike) : Sum  Inputs=+-
  Demux : Demux  Outputs=11
  Icoil1 ref : Subsystem
  Icoil10 ref : Subsystem
  Icoil11 ref : Subsystem
  Icoil2 ref : Subsystem
  Icoil3 ref : Subsystem
  Icoil4 ref : Subsystem
  Icoil5 ref : Subsystem
  Icoil6 ref : Subsystem
  Icoil7 ref : Subsystem
  Icoil8 ref : Subsystem
  Icoil9 ref : Subsystem
  Mux : Mux  Inputs=11
  err Ic : Outport
  wires:
  Icoil_11/1 -> Demux/1
  Demux/1 -> Add3/1
  Icoil2 ref/1(" ") -> Add1/2
  Demux/2 -> Add1/1
  Demux/3 -> Add2/1
  Icoil3 ref/1(" ") -> Add2/2
  Icoil4 ref/1(" ") -> Add4/2
  Demux/4 -> Add4/1
  Icoil5 ref/1(" ") -> Add5/2
  Demux/5 -> Add5/1
  Icoil6 ref/1("  ") -> Add6/2
  Demux/6 -> Add6/1
  Icoil7 ref/1(" ") -> Add7/2
  Demux/7 -> Add7/1
  Icoil8 ref/1("  ") -> Add8/2
  Demux/8 -> Add8/1
  Icoil9 ref/1(" ") -> Add9/2
  Demux/9 -> Add9/1
  Icoil10 ref/1(" ") -> Add10/2
  Demux/10 -> Add10/1
  Icoil11 ref/1(" ") -> Add11/2
  Demux/11 -> Add11/1
  Add3/1 -> Mux/1
  Add1/1 -> Mux/2
  Add2/1 -> Mux/3
  Add4/1 -> Mux/4
  Add6/1 -> Mux/6
  Add7/1 -> Mux/7
  Add8/1 -> Mux/8
  Add9/1 -> Mux/9
  Add10/1 -> Mux/10
  Add11/1 -> Mux/11
  Add5/1 -> Mux/5
  Icoil1 ref/1(" ") -> Add3/2
  eob/1 -> Icoil11 ref/2(eob), Icoil10 ref/2(eob), Icoil9 ref/2(eob), Icoil8 ref/2(eob), Icoil7 ref/2(eob), Icoil6 ref/2(eob), Icoil5 ref/2(eob), Icoil4 ref/2(eob), Icoil3 ref/2(eob), Icoil2 ref/2(eob), Icoil1 ref/2(eob)
  Time/1 -> Icoil5 ref/1(Time), Icoil4 ref/1(Time), Icoil3 ref/1(Time), Icoil2 ref/1(Time), Icoil1 ref/1(Time), Icoil6 ref/1(Time), Icoil7 ref/1(Time), Icoil8 ref/1(Time), Icoil9 ref/1(Time), Icoil10 ref/1(Time), Icoil11 ref/1(Time)
  Mux/1 -> err Ic/1

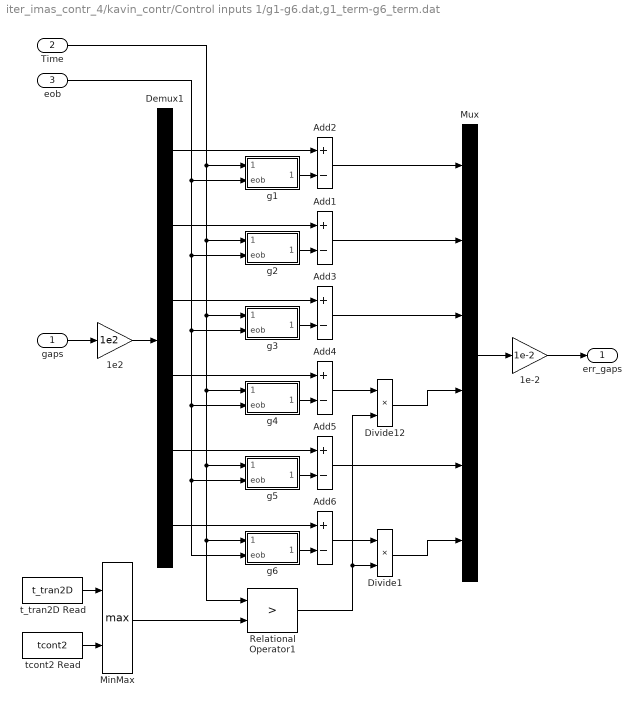
== system iter_imas_contr_4/kavin_contr/Control inputs 1/g1-g6.dat,g1_term-g6_term.dat ==
  gaps : Inport
  Time : Inport  Port=2
  eob : Inport  Port=3
  1e-2 : Gain  Gain=1e-2
  1e2 : Gain  Gain=1e2
  Add{1..6} (6 alike) : Sum  Inputs=+-
  Demux1 : Demux  Outputs=6
  Divide1 : Product  Inputs=**
  Divide12 : Product  Inputs=**
  MinMax : MinMax  Function=max  Inputs=2
  Mux : Mux  Inputs=6
  Relational Operator1 : RelationalOperator  Operator=>  OutDataTypeStr=float('double')
  g1 : Subsystem
  g2 : Subsystem
  g3 : Subsystem
  g4 : Subsystem
  g5 : Subsystem
  g6 : Subsystem
  t_tran2D Read : DataStoreRead  DataStoreName=t_tran2D  DataStoreElements=t_tran2D
  tcont2 Read : DataStoreRead  DataStoreName=tcont2  DataStoreElements=tcont2
  err_gaps : Outport
  wires:
  gaps/1 -> 1e2/1
  Time/1 -> Relational Operator1/1, g6/1(Time), g5/1(Time), g4/1(Time), g3/1(Time), g2/1(Time), g1/1(Time)
  Demux1/1 -> Add2/1
  Demux1/2 -> Add1/1
  g2/1(Out1) -> Add1/2
  g3/1(Out1) -> Add3/2
  Demux1/3 -> Add3/1
  Demux1/4 -> Add4/1
  g4/1(Out1) -> Add4/2
  Demux1/5 -> Add5/1
  g5/1(Out1) -> Add5/2
  Demux1/6 -> Add6/1
  1e2/1 -> Demux1/1
  1e-2/1 -> err_gaps/1
  g1/1(Out1) -> Add2/2
  eob/1 -> g6/2(eob), g5/2(eob), g4/2(eob), g3/2(eob), g2/2(eob), g1/2(eob)
  g6/1(Out1) -> Add6/2
  Mux/1 -> 1e-2/1
  Add2/1 -> Mux/1
  Add1/1 -> Mux/2
  Add5/1 -> Mux/5
  Add4/1 -> Divide12/1
  Divide12/1 -> Mux/4
  Relational Operator1/1 -> Divide1/2, Divide12/2
  Add6/1 -> Divide1/1
  Divide1/1 -> Mux/6
  Add3/1 -> Mux/3
  MinMax/1 -> Relational Operator1/2
  t_tran2D Read/1 -> MinMax/1
  tcont2 Read/1 -> MinMax/2

== system iter_imas_contr_4/kavin_contr/Control inputs 1/trd ==
  time : Inport
  eob : Inport  Port=2
  Ip : Inport  Port=3
  Abs : Abs
  Compare To Constant1 : simulink/Logic and Bit Operations/Compare To Constant  relop=<  const=1  OutDataTypeStr=boolean  ZeroCross=off
  Data Store Read2 : DataStoreRead  DataStoreName=Ip_rd
  "If " : If  NumInputs=2  IfExpression=u1>=1 & u2 >=1  ShowElse=off
  If Action Subsystem2 : Subsystem  TreatAsAtomicUnit=on
  Logical Operator : Logic  Operator=NAND  AllPortsSameDT=off  OutDataTypeStr=float('double')
  Logical Operator1 : Logic  AllPortsSameDT=off  OutDataTypeStr=float('double')
  Memory1 : Memory
  Relational Operator2 : RelationalOperator  Operator=<=  OutDataTypeStr=boolean
  Trigger : Subsystem
  wires:
  Relational Operator2/1 -> Logical Operator1/1
  Data Store Read2/1 -> Abs/1
  Abs/1 -> Relational Operator2/2
  eob/1 -> Compare To Constant1/1
  Logical Operator1/1 -> Trigger/1(Input)
  Compare To Constant1/1 -> Logical Operator1/2
  Memory1/1 -> Logical Operator/2
  "If "/1 -> If Action Subsystem2/Action
  Logical Operator/1 -> "If "/2
  Trigger/1(State) -> "If "/1, Memory1/1, Logical Operator/1
  time/1 -> If Action Subsystem2/1("time ")
  Ip/1 -> Relational Operator2/1

== system iter_imas_contr_4/kavin_contr/Control inputs 1/tterm ==
  Time : Inport
  eob : Inport  Port=2
  Ip : Inport  Port=3
  Compare To Constant1 : simulink/Logic and Bit Operations/Compare To Constant  relop=<  const=1  OutDataTypeStr=boolean  ZeroCross=off
  "If " : If  NumInputs=2  IfExpression=u1>=1 & u2 >=1  ShowElse=off
  If Action Subsystem2 : Subsystem  TreatAsAtomicUnit=on
  Ip<cIp_end : Subsystem
  Logical Operator : Logic  Operator=NAND  AllPortsSameDT=off  OutDataTypeStr=float('double')
  Logical Operator2 : Logic  AllPortsSameDT=off  OutDataTypeStr=float('double')
  Memory1 : Memory
  Trigger : Subsystem
  wires:
  Compare To Constant1/1 -> Logical Operator2/2
  Logical Operator2/1 -> Trigger/1(Input)
  Ip<cIp_end/1(Out1) -> Logical Operator2/1
  Ip/1 -> Ip<cIp_end/1(Ip)
  eob/1 -> Compare To Constant1/1
  Memory1/1 -> Logical Operator/2
  Logical Operator/1 -> "If "/2
  Trigger/1(State) -> Memory1/1, Logical Operator/1, "If "/1
  Time/1 -> If Action Subsystem2/1("time ")
  "If "/1 -> If Action Subsystem2/Action

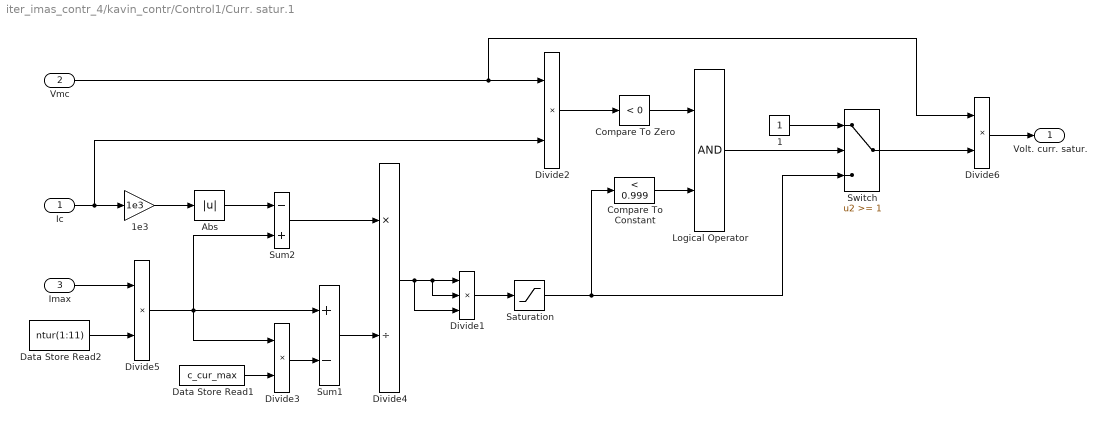
== system iter_imas_contr_4/kavin_contr/Control1/Curr. satur.1 ==
  Ic : Inport
  Vmc : Inport  Port=2
  Imax : Inport  Port=3
  1 : Constant
  1e3 : Gain  Gain=1e3
  Abs : Abs
  Compare To Constant : simulink/Logic and Bit Operations/Compare To Constant  relop=<  const=0.999  OutDataTypeStr=uint8  ZeroCross=off
  Compare To Zero : simulink/Logic and Bit Operations/Compare To Zero  relop=<  OutDataTypeStr=uint8  ZeroCross=off
  Data Store Read1 : DataStoreRead  DataStoreName=c_cur_max  DataStoreElements=c_cur_max
  Data Store Read2 : DataStoreRead  DataStoreName=ntur  DataStoreElements=ntur(1:11)
  Divide1 : Product  Inputs=***
  Divide{2..3,5..6} (4 alike) : Product  Inputs=**
  Divide4 : Product  Inputs=*/
  Logical Operator : Logic  AllPortsSameDT=off  OutDataTypeStr=float('double')
  Saturation : Saturate  UpperLimit=1  LowerLimit=-1
  Sum1 : Sum  Inputs=+-
  Sum2 : Sum  Inputs=-+
  Switch : Switch  Threshold=1
  Volt. curr. satur. : Outport
  wires:
  Ic/1 -> 1e3/1, Divide2/2
  1e3/1 -> Abs/1
  Imax/1 -> Divide5/1
  Abs/1 -> Sum2/1
  Divide5/1 -> Divide3/1, Sum1/1, Sum2/2
  Divide3/1 -> Sum1/2
  Sum2/1 -> Divide4/1
  Sum1/1 -> Divide4/2
  Divide4/1 -> Divide1/1, Divide1/2, Divide1/3
  Divide1/1 -> Saturation/1
  Vmc/1 -> Divide2/1, Divide6/1
  Divide6/1 -> Volt. curr. satur./1
  Saturation/1 -> Switch/3, Compare To Constant/1
  Divide2/1 -> Compare To Zero/1
  Compare To Constant/1 -> Logical Operator/2
  Compare To Zero/1 -> Logical Operator/1
  Switch/1 -> Divide6/2
  Data Store Read1/1 -> Divide3/2
  Data Store Read2/1 -> Divide5/2
  Logical Operator/1 -> Switch/2
  1/1 -> Switch/1

== system iter_imas_contr_4/kavin_contr/Control1/Sum ==
  Lim.contr. : Inport
  Div.contr. : Inport  Port=2
  Curr. term. contr : Inport  Port=3
  volt.dat : Inport  Port=4
  Sum3 : Sum  Inputs=++++
  To Workspace : ToWorkspace  VariableName=Vff_sim  SampleTime=-1
  "  " : Outport
  wires:
  Lim.contr./1 -> Sum3/1
  volt.dat/1 -> To Workspace/1, Sum3/4
  Curr. term. contr/1 -> Sum3/3
  Div.contr./1 -> Sum3/2
  Sum3/1 -> "  "/1

== system iter_imas_contr_4/kavin_contr/Control1/VS control ==
  VS3 err : Inport
  Time : Inport  Port=2
  eob : Inport  Port=3
  Ipl : Inport  Port=4
  Divide10 : Product  Inputs=**
  Ip>cIp_end : Subsystem
  c_eob1 : Switch  Threshold=1
  dzdt noise1 : Subsystem
  eob < 1 : Subsystem
  eob >= 1 : Subsystem
  t_tran2D : Subsystem
  Vvs : Outport
  wires:
  Ipl/1 -> eob >= 1/1(Ipl), eob < 1/2(Ip)
  Time/1 -> eob >= 1/2(time), dzdt noise1/2(Time), t_tran2D/2(Time), eob < 1/4("time "), Ip>cIp_end/1(time)
  eob < 1/1(Out1) -> c_eob1/3
  t_tran2D/1(Out1) -> eob < 1/1(err VS), eob >= 1/3(err VS)
  dzdt noise1/1(Out1) -> t_tran2D/1(Noise,VS3)
  VS3 err/1 -> dzdt noise1/1(VS3 inputs)
  eob >= 1/1(Out1) -> c_eob1/1
  eob/1 -> eob < 1/3("eob "), c_eob1/2
  c_eob1/1 -> Divide10/1
  Ip>cIp_end/1(1 or 0) -> Divide10/2
  Divide10/1 -> Vvs/1

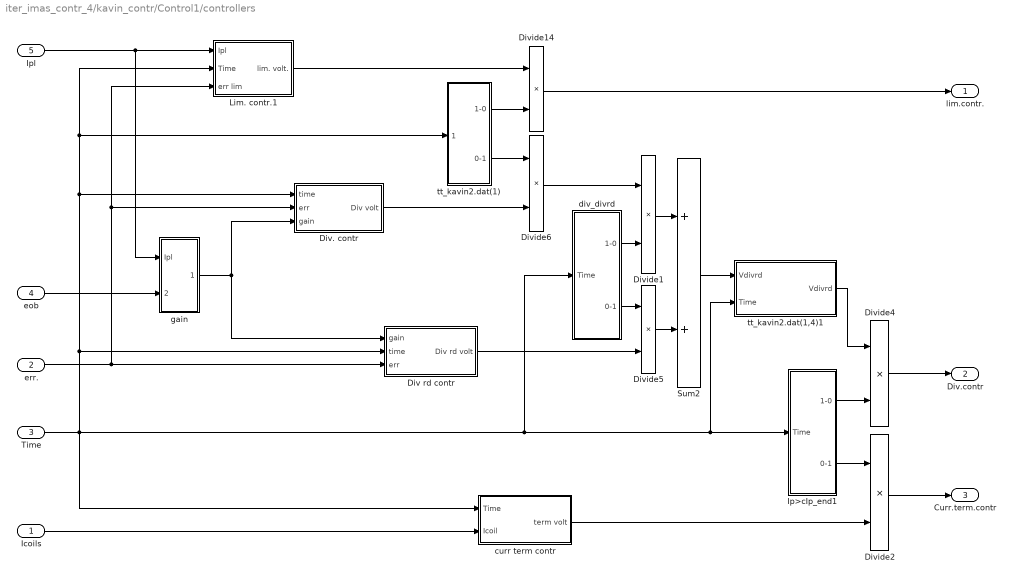
== system iter_imas_contr_4/kavin_contr/Control1/controllers ==
  Icoils : Inport
  err. : Inport  Port=2
  "Time " : Inport  Port=3
  eob : Inport  Port=4
  Ipl : Inport  Port=5
  " tt_kavin2.dat(1)" : Subsystem
  Div rd contr : Subsystem
  Div. contr : Subsystem
  Divide{1..2,4..6,14} (6 alike) : Product  Inputs=**
  Ip>cIp_end1 : Subsystem
  Lim. contr.1 : Subsystem
  Sum2 : Sum
  curr term contr : Subsystem
  div_divrd : Subsystem
  gain : Subsystem
  tt_kavin2.dat(1,4)1 : Subsystem
  lim.contr. : Outport
  Div.contr : Outport  Port=2
  Curr.term.contr : Outport  Port=3
  wires:
  Ipl/1 -> Lim. contr.1/1(Ipl), gain/1(Ipl)
  eob/1 -> gain/2(eob)
  gain/1(Out1) -> Div. contr/3(gain), Div rd contr/1(gain)
  err./1 -> Lim. contr.1/3(err lim), Div. contr/2(err), Div rd contr/3(err)
  div_divrd/1(1-0) -> Divide1/2
  Divide14/1 -> lim.contr./1
  Lim. contr.1/1(lim. volt.) -> Divide14/1
  Divide1/1 -> Sum2/1
  Sum2/1 -> tt_kavin2.dat(1,4)1/1(Vdivrd)
  " tt_kavin2.dat(1)"/1(1-0) -> Divide14/2
  Divide5/1 -> Sum2/2
  div_divrd/2(0-1) -> Divide5/1
  Divide6/1 -> Divide1/1
  " tt_kavin2.dat(1)"/2(0-1) -> Divide6/1
  Div. contr/1("Div volt ") -> Divide6/2
  Div rd contr/1(Div rd volt) -> Divide5/2
  Ip>cIp_end1/2(0-1) -> Divide2/1
  Divide2/1 -> Curr.term.contr/1
  "Time "/1 -> Ip>cIp_end1/1(Time), tt_kavin2.dat(1,4)1/2(Time), div_divrd/1(Time), " tt_kavin2.dat(1)"/1(Time), Lim. contr.1/2(Time), Div. contr/1(time), Div rd contr/2(time), curr term contr/1(Time)
  Icoils/1 -> curr term contr/2(Icoil)
  curr term contr/1(term volt) -> Divide2/2
  tt_kavin2.dat(1,4)1/1("Vdivrd ") -> Divide4/1
  Ip>cIp_end1/1(1-0) -> Divide4/2
  Divide4/1 -> Div.contr/1

== system iter_imas_contr_4/kavin_contr/Control1/volt.dat ==
  Time : Inport
  Divide7 : Product  Inputs=**
  Mux : Mux  Inputs=11
  tterm tr : Subsystem
  volt1 : Subsystem
  volt10 : Subsystem
  volt11 : Subsystem
  volt2 : Subsystem
  volt3 : Subsystem
  volt4 : Subsystem
  volt5 : Subsystem
  volt6 : Subsystem
  volt7 : Subsystem
  volt8 : Subsystem
  volt9 : Subsystem
  volt : Outport
  wires:
  Mux/1 -> Divide7/1
  Time/1 -> tterm tr/1(Time), volt1/1(Time), volt2/1(Time), volt3/1(Time), volt4/1(Time), volt5/1(Time), volt11/1(Time), volt10/1(Time), volt9/1(Time), volt8/1(Time), volt7/1(Time), volt6/1(Time)
  volt1/1(Out1) -> Mux/1
  volt2/1(Out1) -> Mux/2
  volt3/1(Out1) -> Mux/3
  volt4/1(Out1) -> Mux/4
  volt5/1(Out1) -> Mux/5
  volt6/1(Out1) -> Mux/6
  volt7/1(Out1) -> Mux/7
  volt8/1(Out1) -> Mux/8
  volt9/1(Out1) -> Mux/9
  volt10/1(Out1) -> Mux/10
  volt11/1(Out1) -> Mux/11
  Divide7/1 -> volt/1
  tterm tr/1(1 or 0) -> Divide7/2

== system iter_imas_contr_4/kavin_contr/Subsystem1/Subsystem ==
  Zcurr : Inport
  xleft : Inport  Port=2
  xright : Inport  Port=3
  gaps1_6 : Inport  Port=4
  Mux3 : Mux
  Selector : Selector  InputPortWidth=9  Indices=[1 2 7 4 5 8]
  gaps : Outport
  wires:
  gaps1_6/1 -> Mux3/1
  xright/1 -> Mux3/2
  Mux3/1 -> Selector/1
  Selector/1 -> gaps/1
  xleft/1 -> Mux3/3
  Zcurr/1 -> Mux3/4

== system iter_imas_contr_4/kavin_contr/Control inputs 1/Err.1/Trigger ==
  Input : Inport
  Logical Operator : Logic  Operator=OR  AllPortsSameDT=off  OutDataTypeStr=float('double')
  Memory : Memory
  State : Outport
  wires:
  Memory/1 -> Logical Operator/2
  Input/1 -> Logical Operator/1
  Logical Operator/1 -> State/1, Memory/1

== system iter_imas_contr_4/kavin_contr/Control inputs 1/Err.1/tdiv if Ip is set  ==
  1 or 0 : Inport
  "tIp_tr " : Inport  Port=2
  Time : Inport  Port=3
  "If Action " : Subsystem  TreatAsAtomicUnit=on
  Logical Operator : Logic  Operator=NAND  AllPortsSameDT=off  OutDataTypeStr=float('double')
  Memory1 : Memory
  "u1<0 & u2 >=1 & u3>=1 " : If  NumInputs=3  IfExpression=u1<0 & u2 >=1 & u3>=1  ShowElse=off
  wires:
  Time/1 -> "If Action "/1(Time)
  "tIp_tr "/1 -> "u1<0 & u2 >=1 & u3>=1 "/1
  Logical Operator/1 -> "u1<0 & u2 >=1 & u3>=1 "/3
  1 or 0/1 -> "u1<0 & u2 >=1 & u3>=1 "/2, Logical Operator/1, Memory1/1
  "u1<0 & u2 >=1 & u3>=1 "/1 -> "If Action "/Action
  Memory1/1 -> Logical Operator/2

== system iter_imas_contr_4/kavin_contr/Control inputs 1/Ics1_end/Trigger ==
  Input : Inport
  Logical Operator : Logic  Operator=OR  AllPortsSameDT=off  OutDataTypeStr=float('double')
  Memory : Memory
  State : Outport
  wires:
  Memory/1 -> Logical Operator/2
  Input/1 -> Logical Operator/1
  Logical Operator/1 -> State/1, Memory/1

== system iter_imas_contr_4/kavin_contr/Control inputs 1/err(Ic) scr_data.dat/Icoil1 ref ==
  Time : Inport
  eob : Inport  Port=2
  Divide1 : Product  Inputs=**
  I1 : simulink/Lookup Tables/Lookup Table Dynamic  LookUpMeth=Interpolation-Use End Values  OutDataTypeStr=fixdt('double')  OutputDataTypeScalingMode=Specify via dialog  OutDataType=fixdt('double')  OutScaling=2^-10  DoSatur=off
  Memory2 : Memory
  c_eob : Switch  Threshold=1
  scr1 Read : DataStoreRead  DataStoreName=scr_data  DataStoreElements=scr_data(1,:)
  scr2 Read : DataStoreRead  DataStoreName=scr_data  DataStoreElements=scr_data(3,:)
  " " : Outport
  wires:
  c_eob/1 -> Memory2/1, Divide1/1
  Divide1/1 -> " "/1
  Time/1 -> I1/1
  eob/1 -> c_eob/2, Divide1/2
  Memory2/1 -> c_eob/3
  scr2 Read/1 -> I1/3
  I1/1 -> c_eob/1
  scr1 Read/1 -> I1/2

== system iter_imas_contr_4/kavin_contr/Control inputs 1/err(Ic) scr_data.dat/Icoil10 ref ==
  Time : Inport
  eob : Inport  Port=2
  Divide1 : Product  Inputs=**
  I1 : simulink/Lookup Tables/Lookup Table Dynamic  LookUpMeth=Interpolation-Use End Values  OutDataTypeStr=fixdt('double')  OutputDataTypeScalingMode=Specify via dialog  OutDataType=fixdt('double')  OutScaling=2^-10  DoSatur=off
  Memory2 : Memory
  c_eob : Switch  Threshold=1
  scr1 Read : DataStoreRead  DataStoreName=scr_data  DataStoreElements=scr_data(1,:)
  scr12 Read : DataStoreRead  DataStoreName=scr_data  DataStoreElements=scr_data(12,:)
  " " : Outport
  wires:
  c_eob/1 -> Memory2/1, Divide1/1
  Divide1/1 -> " "/1
  Time/1 -> I1/1
  eob/1 -> c_eob/2, Divide1/2
  Memory2/1 -> c_eob/3
  scr12 Read/1 -> I1/3
  I1/1 -> c_eob/1
  scr1 Read/1 -> I1/2

== system iter_imas_contr_4/kavin_contr/Control inputs 1/err(Ic) scr_data.dat/Icoil11 ref ==
  Time : Inport
  eob : Inport  Port=2
  Divide1 : Product  Inputs=**
  I1 : simulink/Lookup Tables/Lookup Table Dynamic  LookUpMeth=Interpolation-Use End Values  OutDataTypeStr=fixdt('double')  OutputDataTypeScalingMode=Specify via dialog  OutDataType=fixdt('double')  OutScaling=2^-10  DoSatur=off
  Memory2 : Memory
  c_eob : Switch  Threshold=1
  scr1 Read : DataStoreRead  DataStoreName=scr_data  DataStoreElements=scr_data(1,:)
  scr13 Read : DataStoreRead  DataStoreName=scr_data  DataStoreElements=scr_data(13,:)
  " " : Outport
  wires:
  c_eob/1 -> Divide1/1, Memory2/1
  Divide1/1 -> " "/1
  Time/1 -> I1/1
  eob/1 -> c_eob/2, Divide1/2
  Memory2/1 -> c_eob/3
  scr13 Read/1 -> I1/3
  I1/1 -> c_eob/1
  scr1 Read/1 -> I1/2
